simulink model "Lab2_AircraftEPS"  (Simulink 8.8)
settings: Solver=ode3  StartTime=0.0  StopTime=10  RelTol=1e-3  EnableMultiTasking=on
PreLoadFcn:
  | warning off
  | Ts=10e-6;
InitFcn:
  | warning off
  | Ts=10e-6;
undefined symbols (not defined in the file): D1, Delta, sigbuilder_block
libraries: powerlib x91, sps_avr x4, powerlib_extras x4, checkVoltage x4
(part 3 of 3)

== stateflow chart BPCU/Chart ==
  state C1 [parallel]
    settings: executionOrder=1
    state On
      entry: B1 = 1
    state Off
      entry: B1 = 0;
    (default) -> C1.Off
    C1.Off -> C1.On : [GL == 1 && in(S.On)]
    C1.On -> C1.Off : [GL==0 && in(S.Off)]
  state C2 [parallel]
    settings: executionOrder=2
    state Off
      entry: B2 = 0;
    state On
      entry: B2 = 1
    C2.Off -> C2.On : [GL == 0 && AL == 1 && !in(C3.On) && in(S.On)]
    (default) -> C2.Off
    C2.On -> C2.Off : [AL==0 && in(S.Off)]
  state C3 [parallel]
    settings: executionOrder=3
    state Off
      entry: B3 = 0;
    state On
      entry: B3 = 1
    (default) -> C3.Off
    C3.Off -> C3.On : [GL == 0 && AR == 1 && !in(C2.On) && in(S.On)]
    C3.On -> C3.Off : [AR==0 && in(S.Off)]
  state C4 [parallel]
    settings: executionOrder=4
    state On
      entry: B4 = 1
    state Off
      entry: B4 = 0;
    (default) -> C4.Off
    C4.Off -> C4.On : [GR == 1 && in(S.On)]
    C4.On -> C4.Off : [GR==0 && in(S.Off)]
  state C5 [parallel]
    settings: executionOrder=5
    state Off
      entry: B5 = 0;
    state On
      entry: B5 = 1
    (default) -> C5.Off
    C5.Off -> C5.On : [(GL == 0 || (GR == 0 && AL == 0 && AR ==0)) && in(S.On)]
  state C6 [parallel]
    settings: executionOrder=6
    state On
      entry: B6= 1
    state Off
      entry: B6 = 0;
    (default) -> C6.Off
    C6.Off -> C6.On : [(GR == 0 || (GL == 0 && AL == 0 && AR ==0)) && in(S.On)]
  state C7 [parallel]
    settings: executionOrder=7
    state On
      entry: B7 = 1
    (default) -> C7.On
  state C8 [parallel]
    settings: executionOrder=8
    state On
      entry: B8 = 1
    (default) -> C8.On
  state C11 [parallel]
    settings: executionOrder=11
    state Off
      entry: B11 = 0;
    (default) -> C11.Off
  state C9 [parallel]
    settings: executionOrder=9
    state On
      entry: B9 = 1
    (default) -> C9.On
  state C12 [parallel]
    settings: executionOrder=12
    state Off
      entry: B12 = 0;
    (default) -> C12.Off
  state C10 [parallel]
    settings: executionOrder=10
    state On
      entry: B10 = 1
    (default) -> C10.On
  state S [parallel]
    settings: executionOrder=13
    state Listen
    state Off
    state On
    S.On -> Listen
    Listen -> S.Off : [hasChanged(GL) || hasChanged(GR) || hasChanged(AL) || hasChanged(AR)]
    (default) -> S.Off
    S.Off -> S.On
  data: B1 output double; GL input double; B2 output double; B3 output double; B4 output double; B5 output double; B6 output double; B7 output double; B8 output double; B9 output double; B10 output double; B11 output double; B12 output double; GR input double; AL input double; AR input double
  events: tick input RISING_EDGE_EVENT
